simulink model "simulare_bucla_deschisa"  (R2023b)
settings: Solver=VariableStepAuto  StartTime=0.0  StopTime=20  RelTol=1e-3
values from neighbouring files (symbols this model uses):
  A = [0 lambda 0 0 ... (first row only)    [rotary_inverted_pendulum.m]    (also in sis_liniar.m)
  B = [0; B21; 0; B41]./lambda    [rotary_inverted_pendulum.m]    (also in sis_liniar.m)
  initialConditions = [1;1;1;1]    [rotary_inverted_pendulum.m]
  stepFinalValue = 1    [rotary_inverted_pendulum.m]
settings Model: Creator=ovidiuceoca  LastModifiedBy=ovidiuceoca

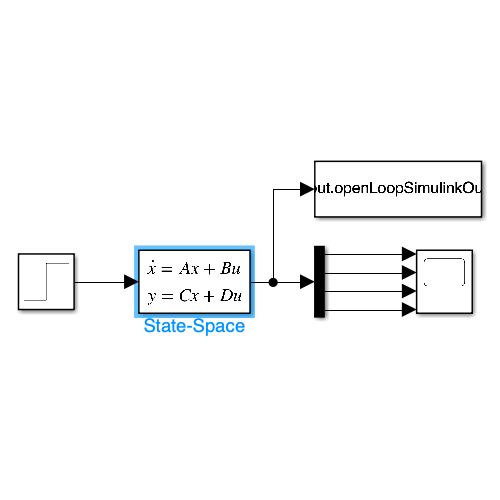
[thumbnail: Simulink's stored preview of the top-level diagram]
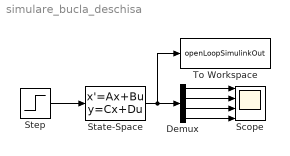
== system simulare_bucla_deschisa ==
  Demux : Demux
  Scope : Scope  NumInputPorts=4
  State-Space : StateSpace  A=A  B=B  C=eye(4)  D=[0;0;0;0]  InitialCondition=initialConditions
  Step : Step  Time=0  After=stepFinalValue  SampleTime=0
  To Workspace : ToWorkspace  VariableName=openLoopSimulinkOut  SaveFormat=Timeseries  SampleTime=-1
  wires:
  Step/1 -> State-Space/1
  State-Space/1 -> To Workspace/1, Demux/1
  Demux/2 -> Scope/2
  Demux/1 -> Scope/1
  Demux/3 -> Scope/3
  Demux/4 -> Scope/4
